simulink model "Supercapacitor"  (R2024b)
settings: Solver=VariableStepAuto  StartTime=0.0  StopTime=10.0  RelTol=1e-3
libraries: spsSeriesRLCBranchLib x7, spsControlledCurrentSourceLib x1, spsCurrentMeasurementLib x1, spsVoltageMeasurementLib x1, sps_lib x1
settings Model: Creator=holthoff  LastModifiedBy=holthoff

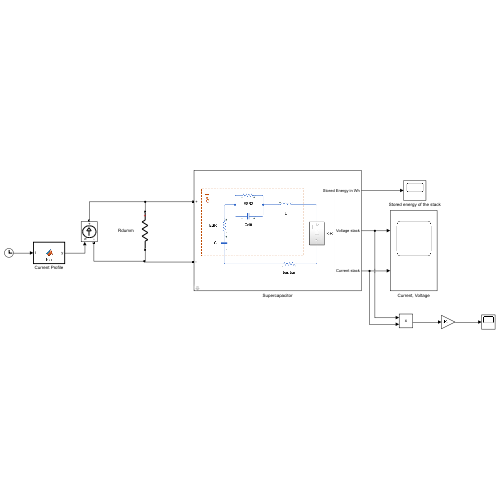
[thumbnail: Simulink's stored preview of the top-level diagram]
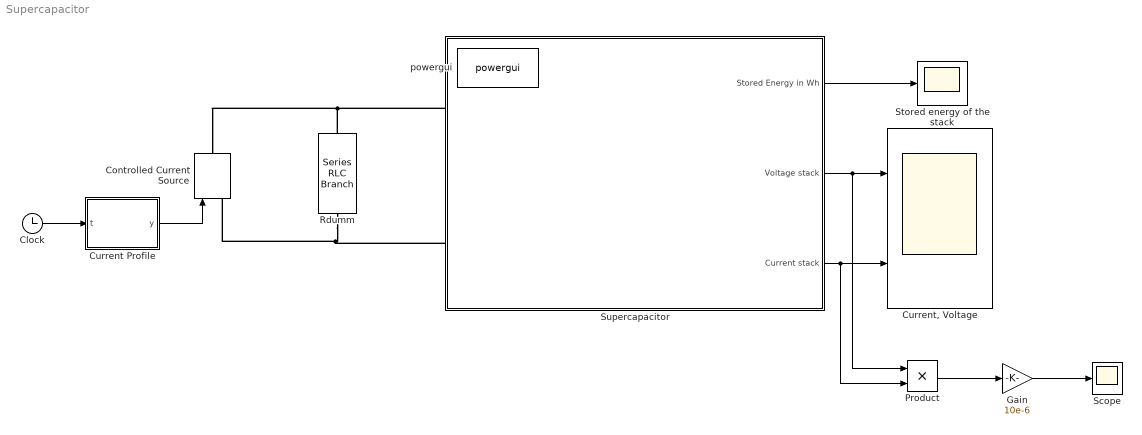
== system Supercapacitor ==
  Clock : Clock
  Controlled Current Source : spsControlledCurrentSourceLib/Controlled Current Source  Initialize=on  Source_Type=AC  Amplitude=0  Phase=0  Frequency=0  Measurements=None
  Current Profile : MATLAB Function  TreatAsAtomicUnit=on
  "Current, Voltage" : Scope  NumInputPorts=2
  Gain : Gain  Gain=10e-6
  Product : Product
  Rdumm : spsSeriesRLCBranchLib/Series RLC Branch  LConnTagsString=__new0  RConnTagsString=__new0  BranchType=R  Resistance=100  Inductance=1e-3  SetiL0=off  InitialCurrent=0  Capacitance=1e-6  Setx0=off  InitialVoltage=0  Measurements=None
  Scope : Scope
  Stored energy of the stack : Scope
  Supercapacitor : Subsystem  mask{C1=2560, R3=0.00014, R4=4e-05, Cdiff1=750, num_cells=55, V_init=125/55, I_init=0, Rbus=3e-05}
      mask prompts: C1 "Capacitance C (F)"; R3 "Equivalent Series Resistance (Ohm)"; R4 "Equivalent Series Resistance 2 (Ohm)"; Cdiff1 "Capacitance Cdiff (F)"; num_cells "Number of cells in series"; V_init "Initial Voltage per Capacitor (V)"; I_init "Initial Current of the Inductor (A)"; Rbus "Resistance bus (Ohm)"
      mask DialogControl DescTextVar Prompt: Supercapacitor
      mask DialogControl Control2 Prompt: This generic model represents a supercapacitor stack consisting of an arbitrary number of cells connected in series. The model is designed to simulate the electrical characteristics of the stack, including current, voltage, and stored energy.
      mask DialogControl Control3 Prompt: Copyright © by Fraunhofer IWES
      mask Display: image('SC.png', [10,0,60,0,100,100]);
  powergui : sps_lib/powergui  Priority=1  SimulationMode=Continuous  SampleTime=50e-6  frequency=60  Iterations=50  frequencyindice=0  Pbase=100e6  ErrMax=1e-4  UnitsV=kV  UnitsW=MW  buscounter=0  FunctionMessages=off  echomessages=off  EnableUseOfTLC=off  CurrentSourceSwitches=off  DisableSnubberDevices=off  DisableRonSwitches=off  DisableVfSwitches=off  DisplayEquations=off  AutomaticDiscreteSolvers=off  SolverType=Tustin/Backward Euler (TBE)  Interpol=off  ExternalGateDelay=off  methode=off  Ts=100  x0status=blocks  SPID=on  SwTol=0  HookPort=off  NonlinearTolerance=1e-4  nMaxIteration=100  ContinueOnMaxIteration=off  RestoreLinks=warning  ResistiveCurrentMeasurement=off  Frange=[0:2:500]  Ylog=off  Xlog=on  ShowGrid=off  save=off  variable=ZData  structure=0  ZoomFFT=off  StartTime=0.0  cycles=1  DisplayStyle=1  fundamental=60  FreqAxis=off  MaxFrequency=1000  frequencyindicesteady=1  RmsSteady=1  display=off
  wires:
  Supercapacitor/1(Stored Energy in Wh) -> Stored energy of the stack/1
  Supercapacitor/2(Voltage stack) -> Product/1, "Current, Voltage"/1
  Supercapacitor/3(Current stack) -> Product/2, "Current, Voltage"/2
  Clock/1 -> Current Profile/1(t)
  Current Profile/1(y) -> Controlled Current Source/1
  Product/1 -> Gain/1
  Gain/1 -> Scope/1
  connections:
  Supercapacitor/LConn2 -- Rdumm/RConn1 -- Controlled Current Source/LConn1
  Supercapacitor/LConn1 -- Rdumm/LConn1 -- Controlled Current Source/RConn1

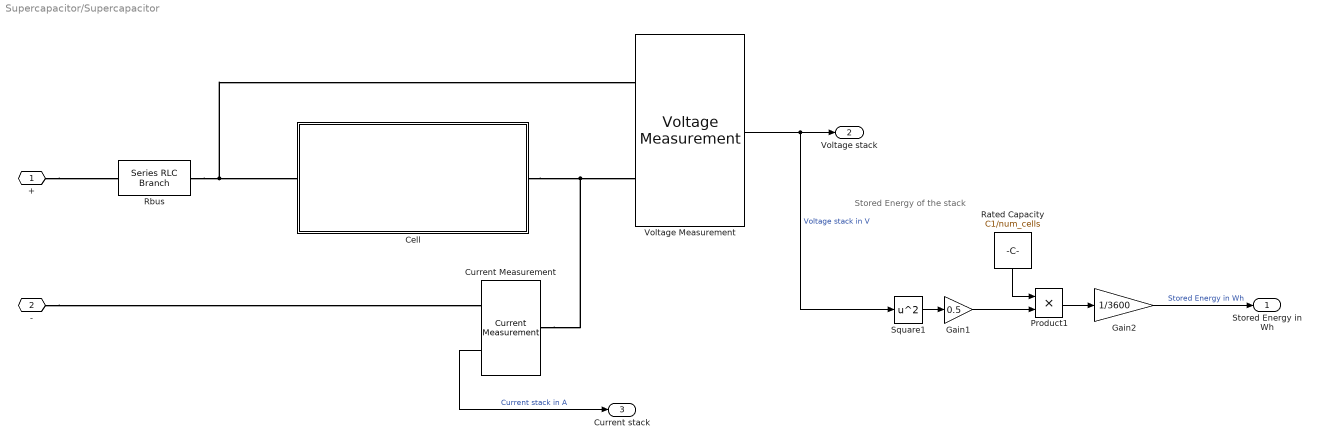
== system Supercapacitor/Supercapacitor ==
  note: Stored Energy of the stack
  Cell : Subsystem
  Current Measurement : spsCurrentMeasurementLib/Current Measurement  PhasorSimulation=off  OutputType=Complex  PSBequivalent=0
  Gain1 : Gain  Gain=0.5
  Gain2 : Gain  Gain=1/3600
  Product1 : Product
  Rated Capacity : Constant  Value=C1/num_cells
  Rbus : spsSeriesRLCBranchLib/Series RLC Branch  LConnTagsString=__new0  RConnTagsString=__new0  BranchType=R  Resistance=Rbus  Inductance=1e-3  SetiL0=off  InitialCurrent=0  Capacitance=1e-6  Setx0=off  InitialVoltage=0  Measurements=None
  Square1 : Math  Operator=square
  Voltage Measurement : spsVoltageMeasurementLib/Voltage Measurement  PhasorSimulation=off  OutputType=Complex  PSBequivalent=0
  + : PMIOPort  Side=Left
  - : PMIOPort  Port=2  Side=Left
  Stored Energy in Wh : Outport
  Voltage stack : Outport  Port=2
  Current stack : Outport  Port=3
  wires:
  Voltage Measurement/1 -> Voltage stack/1, Square1/1  "Voltage stack in V"
  Square1/1 -> Gain1/1
  Current Measurement/1 -> Current stack/1  "Current stack in A"
  Gain2/1 -> Stored Energy in Wh/1  "Stored Energy in Wh"
  Product1/1 -> Gain2/1
  Rated Capacity/1 -> Product1/1
  Gain1/1 -> Product1/2
  connections:
  Current Measurement/LConn1 -- Cell/RConn1 -- Voltage Measurement/LConn2
  Rbus/RConn1 -- Voltage Measurement/LConn1 -- Cell/LConn1
  +/RConn1 -- Rbus/LConn1
  -/RConn1 -- Current Measurement/RConn1

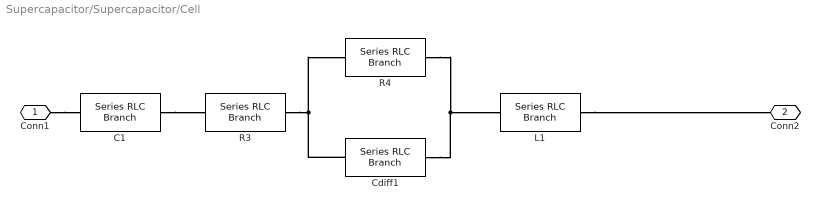
== system Supercapacitor/Supercapacitor/Cell ==
  C1 : spsSeriesRLCBranchLib/Series RLC Branch  LConnTagsString=__new0  RConnTagsString=__new0  BranchType=C  Resistance=1  Inductance=1e-3  SetiL0=off  InitialCurrent=0  Capacitance=C1/num_cells  Setx0=on  InitialVoltage=V_init  Measurements=None
  Cdiff1 : spsSeriesRLCBranchLib/Series RLC Branch  LConnTagsString=__new0  RConnTagsString=__new0  BranchType=C  Resistance=1  Inductance=1e-3  SetiL0=off  InitialCurrent=0  Capacitance=Cdiff1/num_cells  Setx0=on  InitialVoltage=V_init  Measurements=None
  L1 : spsSeriesRLCBranchLib/Series RLC Branch  LConnTagsString=__new0  RConnTagsString=__new0  BranchType=L  Resistance=1  Inductance=3e-08  SetiL0=on  InitialCurrent=I_init  Capacitance=1e-6  Setx0=off  InitialVoltage=0  Measurements=None
  R3 : spsSeriesRLCBranchLib/Series RLC Branch  LConnTagsString=__new0  RConnTagsString=__new0  BranchType=R  Resistance=R3*num_cells  Inductance=1e-3  SetiL0=off  InitialCurrent=0  Capacitance=1e-6  Setx0=off  InitialVoltage=0  Measurements=None
  R4 : spsSeriesRLCBranchLib/Series RLC Branch  LConnTagsString=__new0  RConnTagsString=__new0  BranchType=R  Resistance=R4*num_cells  Inductance=1e-3  SetiL0=off  InitialCurrent=0  Capacitance=1e-6  Setx0=off  InitialVoltage=0  Measurements=None
  Conn1 : PMIOPort  Side=Left
  Conn2 : PMIOPort  Port=2  Side=Right
  connections:
  Conn1/RConn1 -- C1/LConn1
  Cdiff1/LConn1 -- R4/LConn1 -- R3/RConn1
  Cdiff1/RConn1 -- R4/RConn1 -- L1/LConn1
  C1/RConn1 -- R3/LConn1
  L1/RConn1 -- Conn2/RConn1

== matlab function Supercapacitor/Current Profile ==
  data: t input; y output
function y = fcn(t)
    ts = 0.001; % s
    t0 = 0;     % s
    tend = 5;   % s

    if t < t0 || t > tend
        y = 0; 
        return;
    end

    ms1 = 1.99; % s
    ms2 = 2;
    ms3 = 3;
    ms4 = 3.01;

    interval1 = t >= t0 && t < ms1;
    interval2 = t >= ms1 && t < ms2;
    interval3 = t >= ms2 && t < ms3;
    interval4 = t >= ms3 && t < ms4;
    interval5 = t >= ms4 && t <= tend;

    fvseg1 = 0;     % Final value of interval
    fvseg2 = 2202;  % Rated maximum current peak current for 1 s in A
    fvseg3 = 2202;
    fvseg4 = 0;
    fvseg5 = 0;

    if interval1
        y = fvseg1; 
    elseif interval2
        % Ramp up
        y = fvseg1 + (fvseg2 - fvseg1) * ((t - ms1) / (ms2 - ms1));
    elseif interval3
        y = fvseg3; 
    elseif interval4
        % Ramp down
        y = fvseg3 + (fvseg4 - fvseg3) * ((t - ms3) / (ms4 - ms3));
    else
        y = fvseg5;
    end
end
